simulink model "A2_24"  (R2021a)
settings: Solver=VariableStepAuto  StartTime=0.0  StopTime=10.0  RelTol=1e-3
settings Model: Creator=Nils Kutter  LastModifiedBy=Nils Kutter

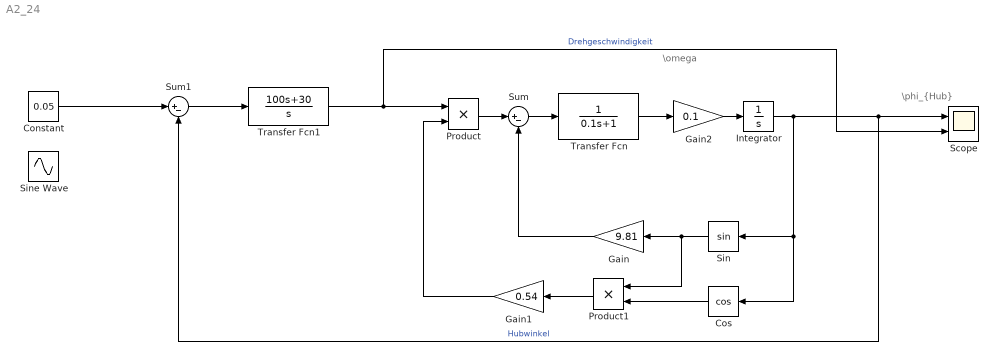
== system A2_24 ==
  note: \phi_{Hub}
  note: \omega
  Constant : Constant  Value=0.05
  Cos : Trigonometry  Operator=cos
  Gain : Gain  Gain=9.81
  Gain1 : Gain  Gain=0.54
  Gain2 : Gain  Gain=0.1
  Integrator : Integrator  InitialCondition=0.01
  Product : Product  RndMeth=Zero
  Product1 : Product  RndMeth=Zero
  Scope : Scope  NumInputPorts=2
  Sin : Trigonometry
  Sine Wave : Sin  Amplitude=0.5  Bias=0.8  SampleTime=0
  Sum : Sum  Inputs=|+-
  Sum1 : Sum  Inputs=|+-
  Transfer Fcn : TransferFcn  Denominator=[0.1 1]
  Transfer Fcn1 : TransferFcn  Numerator=[100 30]  Denominator=[1 0]
  wires:
  Sum1/1 -> Transfer Fcn1/1
  Constant/1 -> Sum1/1
  Transfer Fcn1/1 -> Scope/2, Product/1  "Drehgeschwindigkeit"
  Gain2/1 -> Integrator/1
  Cos/1 -> Product1/2
  Integrator/1 -> Cos/1, Sin/1, Scope/1, Sum1/2  "Hubwinkel"
  Sin/1 -> Gain/1, Product1/1
  Gain1/1 -> Product/2
  Product1/1 -> Gain1/1
  Sum/1 -> Transfer Fcn/1
  Product/1 -> Sum/1
  Gain/1 -> Sum/2
  Transfer Fcn/1 -> Gain2/1
